simulink model "SeaPort"  (R2023b)
(part 2 of 3)

  Aveiro_Sea_Port (61)/4 -> SAVE_11 (11)/1, Display3/1, [CELL_QoS]  "CELL_QoS"
  MOBILE_1 (147)/1 -> SAVE_9 (9)/1, Display8/1, [MOBILE_QoS]  "MOBILE_QoS"
  PowerGen_1 (46)/1 -> ANTENNA_1 (56)/3, ONU_1 (55)/3  "POWER"
  PowerGen_2 (47)/1 -> ONU_2 (58)/3, ANTENNA_2 (60)/3  "POWER"
  PowerGen_3 (157)/1 -> ASR9006_3 (87)/4, [POWER_1], ROOM_1 (51)/1  "POWER"
  PowerGen_4 (214)/1 -> ASR9006_4 (88)/4, [POWER_2], ROOM_2 (52)/1  "POWER"
  ROOM_1 (51)/1 -> ASR9006_3 (87)/5, [ROOM_QoS_1]  "ROOM_QoS"
  ROOM_2 (52)/1 -> ASR9006_4 (88)/5, [ROOM_QoS_2]  "ROOM_QoS"
  [POWER_2] -> ASR903_4 (90)/4  "POWER"
  [ROOM_QoS_2] -> ASR903_4 (90)/5  "ROOM_QoS"
  [POWER_2] -> ASR920_4 (86)/4  "POWER"
  [ROOM_QoS_2] -> ASR920_4 (86)/5  "ROOM_QoS"
  [POWER_2] -> Nex_4 (93)/4  "POWER"
  [ROOM_QoS_2] -> Nex_4 (93)/5  "ROOM_QoS"
  [POWER_2] -> OLT_2 (57)/4  "POWER"
  [ROOM_QoS_2] -> OLT_2 (57)/5  "ROOM_QoS"
  Wire_14b (43)/4 -> Wire_14 (42)/4  "MECH_FAULT"
  Wire_14 (42)/4 -> Wire_14b (43)/4  "MECH_FAULT"
  [POWER_1] -> ASR920_3 (85)/4  "POWER"
  [ROOM_QoS_1] -> ASR920_3 (85)/5  "ROOM_QoS"
  [POWER_1] -> ASR903_3 (89)/4  "POWER"
  [ROOM_QoS_1] -> ASR903_3 (89)/5  "ROOM_QoS"
  [POWER_1] -> OLT_1 (25)/4  "POWER"
  [ROOM_QoS_1] -> OLT_1 (25)/5  "ROOM_QoS"
  Splitter_1 (54)/4 -> OLT_1 (25)/6  "NGPON_IN"
  Splitter_1 (54)/2 -> ONU_2 (58)/2  "CYBER_FAULT"
  Splitter_1 (54)/3 -> ONU_2 (58)/4  "NGPON_CONN"
  Wire_6b (18)/4 -> Wire_6 (17)/4  "MECH_FAULT"
  ASR920_3 (85)/4 -> [Routing_QoS_920_3]  "ROUTING_QoS"
  ASR9006_3 (87)/4 -> [Routing_QoS_9006_3]  "ROUTING_QoS"
  Nex_3 (92)/4 -> [Switching_QoS_Nex_3]  "SWITCHING_QoS"
  ASR903_3 (89)/4 -> [Routing_QoS_903_3]  "ROUTING_QoS"
  [POWER_1] -> Nex_3 (92)/4  "POWER"
  [ROOM_QoS_1] -> Nex_3 (92)/5  "ROOM_QoS"
  Nex_4 (93)/4 -> [Switching_QoS_Nex_4]  "SWITCHING_QoS"
  ASR9006_4 (88)/4 -> [Routing_QoS_9006_2]  "ROUTING_QoS"
  ASR903_4 (90)/4 -> [Routing_QoS_903_4]  "ROUTING_QoS"
  ASR920_4 (86)/4 -> [Routing_QoS_920_4]  "ROUTING_QoS"
  OLT_1 (25)/4 -> Splitter_1 (54)/3  "NGPON_CONN"
  Wire_6 (17)/1 -> ASR9006_3 (87)/1  "TLC_CONN"
  Wire_6 (17)/2 -> ASR9006_3 (87)/2  "TLC_SERVICE"
  Wire_6 (17)/3 -> ASR9006_3 (87)/3  "CYBER_FAULT"
  5G_Core_1 (198)/1 -> TLC_conn9/1  "TLC_CONN"
  5G_Core_1 (198)/2 -> TLC_service9/1  "TLC_SERVICE"
  Alcatel_3 (83)/2 -> Wire_10b (31)/2, 5G_Core_1 (198)/2  "TLC_SERVICE"
  PowerGen_5 (236)/1 -> Alcatel_3 (83)/4, Room_6 (241)/1, 5G_Core_1 (198)/4  "POWER"
  Alcatel_3 (83)/1 -> Wire_10b (31)/1, 5G_Core_1 (198)/1  "TLC_CONN"
  5G_Core_1 (198)/3 -> CYBER_fault9/1  "CYBER_FAULT"
  Alcatel_3 (83)/3 -> Wire_10b (31)/3, 5G_Core_1 (198)/3  "CYBER_FAULT"
  Room_6 (241)/1 -> 5G_Core_1 (198)/5, Building_3 (215)/1, Alcatel_3 (83)/5  "ROOM_QoS"
  CYBER_fault9/1 -> Alcatel_3 (83)/3  "CYBER_FAULT"
  TLC_conn9/1 -> Alcatel_3 (83)/1  "TLC_CONN"
  TLC_service9/1 -> Alcatel_3 (83)/2  "TLC_SERVICE"
  Alcatel_3 (83)/4 -> [Routing_QoS_Alcatel_3]  "ROUTING_QoS"
  Wire_10 (30)/1 -> TLC_conn9/2  "TLC_CONN"
  Wire_10 (30)/2 -> TLC_service9/2  "TLC_SERVICE"
  Wire_10 (30)/3 -> CYBER_fault9/2  "CYBER_FAULT"
  ANTENNA_2 (60)/4 -> [RF_QoS_2], Display4/1  "RF_QoS"
  Nex_3 (92)/2 -> Subsystem/1(TLC_SERVICE)  "TLC_SERVICE"
  Subsystem/1(1) -> R_Wire_1b (99)/2  "TLC_SERVICE"
  Subsystem/3(3) -> TLC_service3/1  "TLC_SERVICE"
  Subsystem/4(4) -> TLC_service4/1  "TLC_SERVICE"
  Subsystem/2(2) -> Wire_8 (21)/2  "TLC_SERVICE"
  Subsystem10/1(MEAN) -> SAVE_8 (8)/1  "GLOBAL_QoS"
  [Switching_QoS_Nex_3] -> Subsystem7/1(1)
  Redundancy/1 -> SAVE_7 (7)/1, Subsystem10/1(1)  "REDUNDANCY_QoS"
  media2/1(y) -> SAVE_5 (5)/1, Subsystem8/2(2)  "ROUTING_QoS"
  [Routing_QoS_9006_3] -> Mux/1
  [RF_QoS_2] -> Subsystem5/2(2)
  [Building_QoS_1] -> SAVE_3 (3)/1  "BUILDING_QoS"
  [MOBILE_QoS] -> Subsystem5/3(3)
  [Routing_QoS_9006_2] -> Mux/2
  Firewall/1 -> SAVE_1 (1)/1  "FIREWALL_GLOBAL_QoS"
  Subsystem7/1(MEAN) -> SAVE_6 (6)/1, Subsystem8/1(1)  "SWITCHING_QoS"
  Subsystem5/1(MEAN) -> SAVE_2 (2)/1, Subsystem10/3(3)  "SERVICES_QoS"
  Subsystem8/1(MEAN) -> SAVE_4 (4)/1, Subsystem10/2(2)  "MPLS_NET_QoS"
  [Routing_QoS_920_4] -> Mux/6
  [RF_QoS_1] -> Subsystem5/1(1)
  Mux/1 -> media2/1(u)
  [Routing_QoS_903_4] -> Mux/4
  [Switching_QoS_Nex_4] -> Subsystem7/2(2)
  [Routing_QoS_903_3] -> Mux/3
  [Routing_QoS_Alcatel_3] -> Mux/7
  [Routing_QoS_920_3] -> Mux/5
  ANTENNA_1 (56)/4 -> Display7/1, [RF_QoS_1]  "RF_QoS"
  [CELL_QoS] -> Subsystem5/4(4)
  Max/1 -> media4/1(u)
  media9/1(y) -> SAVE_20 (20)/1  "ALT_ROUTING"
  media3/1(y) -> SAVE_21 (21)/1  "ALT_SERVICES"
  media4/1(y) -> SAVE_22 (22)/1  "ALT_ALL"
  [Mobile_Alt_Route_1] -> media9/1(u), Display15/1, Max/1
  [Mobile_Alt_Serv_1] -> media3/1(u), Display16/1, Max/2
  MOBILE_1 (147)/2 -> [Mobile_Alt_Route_1]  "ALT_ROUTING"
  MOBILE_1 (147)/3 -> [Mobile_Alt_Serv_1]  "ALT_SERVICES"
  Building_3 (215)/2 -> [Building_QoS_1]  "BUILDING_QoS"
  CISIA_MASTER (0)/4 -> Display21/1  "TIME PAST"
  CISIA_MASTER (0)/2 -> Display11/1  "MAJOR HITS"
  CISIA_MASTER (0)/1 -> Display18/1  "MINOR HITS"
  CISIA_MASTER (0)/3 -> Display20/1  "DELTA TIME"
